simulink model "pmsm_nl_portable"  (R2016a)
settings: Solver=VariableStepAuto  SolverMode=SingleTasking  StartTime=0.0  StopTime=simParam.stopTime  MaxStep=simParam.maxStep  RelTol=1e-3
values from neighbouring files (symbols this model uses):
  b = 0.01    [trim_pmsm.m]
  J = X1_dot^2 + X2_dot^2 + X3_dot^2    [nonLinearPMSMCost.m]    (also in trim_pmsm.m = 0.1)
  lambdaM = 0.14    [trim_pmsm.m]
  Ld = 0.9    [trim_pmsm.m]
  Lq = 0.9    [trim_pmsm.m]
  N = 18    [trim_pmsm.m]
  Rs = 1.3    [trim_pmsm.m]
undefined symbols (not defined in the file or in its folder): simParam, X_i
settings Model: Creator=kaike  LastModifiedBy=kaike
settings DataIOCC: ReturnWorkspaceOutputs=on
settings DebuggingCC: UnconnectedInputMsg=none  UnconnectedOutputMsg=none  UnconnectedLineMsg=none  SFUnexpectedBacktrackingDiag=error  SFNoUnconditionalDefaultTransitionDiag=error
settings ModelReferenceCC: EnableRefExpFcnMdlSchedulingChecks=off
settings SFSimCC: SimUseLocalCustomCode=on
settings RTWCC: Description=Generic Real-Time Target  RTWUseLocalCustomCode=on
settings GRTTargetCC: TargetLangStandard=C99 (ISO)
settings ConfigComp: CovMetricSettings=dwe  CovSaveCumulativeToWorkspaceVar=off  CovSaveSingleToWorkspaceVar=off  CovExternalEMLEnable=on

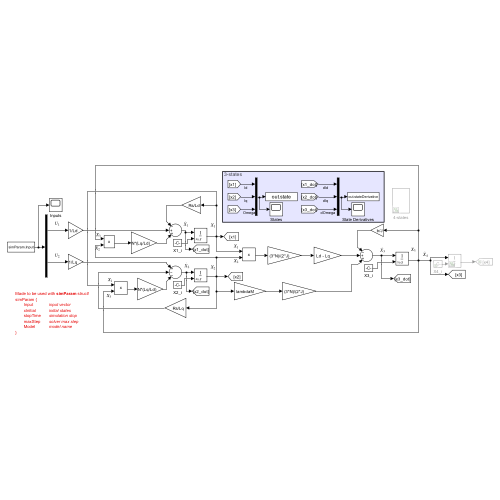
[thumbnail: Simulink's stored preview of the top-level diagram]
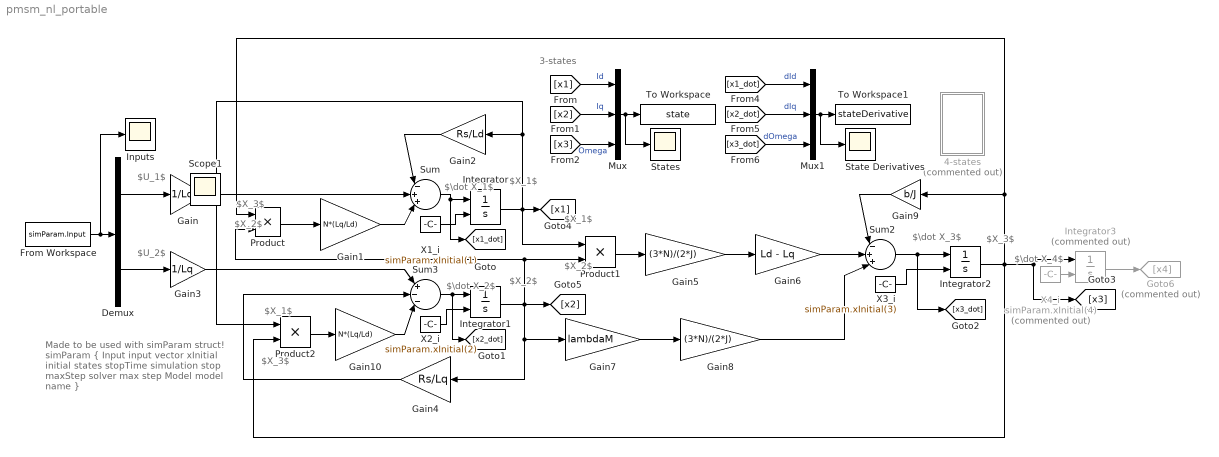
== system pmsm_nl_portable ==
  note: Made to be used with simParam struct!
      | simParam {
      | Input input vector
      | xInitial initial states
      | stopTime simulation stop
      | maxStep solver max step
      | Model model name
      | }
  note: $\dot X_4$
  note: $X_3$
  note: $X_2$
  note: $X_1$
  note: $U_2$
  note: $U_1$
  note: $\dot X_3$
  note: $\dot X_2$
  note: $\dot X_1$
  note: $X_1$
  note: $X_1$
  note: $X_3$
  note: $X_3$
  note: $X_2$
  note: $X_2$
  note: 3-states
  4-states : Subsystem  Commented=on
  Demux : Demux  Outputs=2
  From Workspace : FromWorkspace  VariableName=simParam.Input  OutputAfterFinalValue=Holding final value
  Gain : Gain  Gain=1/Ld
  Gain1 : Gain  Gain=N*(Lq/Ld)
  Gain10 : Gain  Gain=N*(Lq/Ld)
  Gain2 : Gain  Gain=Rs/Ld
  Gain3 : Gain  Gain=1/Lq
  Gain4 : Gain  Gain=Rs/Lq
  Gain5 : Gain  Gain=(3*N)/(2*J)
  Gain6 : Gain  Gain=Ld - Lq
  Gain7 : Gain  Gain=lambdaM
  Gain8 : Gain  Gain=(3*N)/(2*J)
  Gain9 : Gain  Gain=b/J
  Goto6 : Goto  Commented=on  GotoTag=x4
  Inputs : Scope
  Integrator : Integrator  InitialConditionSource=external  InitialCondition=simParam.X_initial(3)  ContinuousStateAttributes='Id'
  Integrator1 : Integrator  InitialConditionSource=external  InitialCondition=X_i(2)  ContinuousStateAttributes='Iq'
  Integrator2 : Integrator  InitialConditionSource=external  InitialCondition=10  ContinuousStateAttributes='omega'
  Integrator3 : Integrator  Commented=on  InitialConditionSource=external  InitialCondition=X_i(4)  ContinuousStateAttributes='theta'
  Mux : Mux  Inputs=3
  Mux1 : Mux  Inputs=3
  Product : Product
  Product1 : Product
  Product2 : Product
  State Derivatives : Scope
  States : Scope
  Sum : Sum  Inputs=|-++|
  Sum2 : Sum  Inputs=|-++|
  Sum3 : Sum  Inputs=|+--|
  To Workspace : ToWorkspace  VariableName=state  SampleTime=-1
  To Workspace1 : ToWorkspace  VariableName=stateDerivative  SampleTime=-1
  X1_i : Constant  Value=simParam.xInitial(1)  VectorParams1D=off
  X2_i : Constant  Value=simParam.xInitial(2)
  X3_i : Constant  Value=simParam.xInitial(3)
  X4_i : Constant  Commented=on  Value=simParam.xInitial(4)
  Scope1 : Scope
  wires:
  From Workspace/1 -> Inputs/1, Demux/1
  Demux/1 -> Gain/1
  Demux/2 -> Gain3/1
  Sum/1 -> [x1_dot], Integrator/1
  Integrator/1 -> [x1], Product2/1, Gain2/1, Product1/1
  Gain2/1 -> Sum/1
  Gain/1 -> Sum/2
  Gain1/1 -> Sum/3
  Gain3/1 -> Sum3/1
  Sum3/1 -> [x2_dot], Integrator1/1
  Integrator1/1 -> [x2], Product/2, Product1/2, Gain4/1, Gain7/1
  Gain4/1 -> Sum3/2
  Product1/1 -> Gain5/1
  Gain5/1 -> Gain6/1
  Gain6/1 -> Sum2/2
  Gain7/1 -> Gain8/1
  Integrator2/1 -> Gain9/1, Product/1, [x3], Integrator3/1, Product2/2
  Gain9/1 -> Sum2/1
  Gain8/1 -> Sum2/3
  Sum2/1 -> [x3_dot], Integrator2/1
  Product/1 -> Gain1/1
  Gain10/1 -> Sum3/3
  Product2/1 -> Gain10/1
  X2_i/1 -> Integrator1/2
  X3_i/1 -> Integrator2/2
  X4_i/1 -> Integrator3/2
  X1_i/1 -> Integrator/2
  Integrator3/1 -> Goto6/1
  [x3_dot] -> Mux1/3  "dOmega"
  [x2] -> Mux/2  "Iq"
  [x1_dot] -> Mux1/1  "dId"
  Mux1/1 -> State Derivatives/1, To Workspace1/1
  [x1] -> Mux/1  "Id"
  [x2_dot] -> Mux1/2  "dIq"
  [x3] -> Mux/3  "Omega"
  Mux/1 -> States/1, To Workspace/1

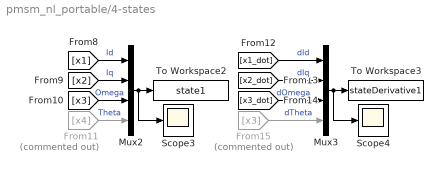
== system pmsm_nl_portable/4-states ==
  From11 : From  Commented=on  GotoTag=x4
  From15 : From  Commented=on  GotoTag=x3
  Mux2 : Mux
  Mux3 : Mux
  Scope3 : Scope
  Scope4 : Scope
  To Workspace2 : ToWorkspace  VariableName=state1  SampleTime=-1
  To Workspace3 : ToWorkspace  VariableName=stateDerivative1  SampleTime=-1
  wires:
  Mux3/1 -> Scope4/1, To Workspace3/1
  [x2] -> Mux2/2  "Iq"
  Mux2/1 -> Scope3/1, To Workspace2/1
  [x3_dot] -> Mux3/3  "dOmega"
  From11/1 -> Mux2/4  "Theta"
  [x3] -> Mux2/3  "Omega"
  [x1] -> Mux2/1  "Id"
  [x1_dot] -> Mux3/1  "dId"
  From15/1 -> Mux3/4  "dTheta"
  [x2_dot] -> Mux3/2  "dIq"
